simulink model "model_monocykl"  (R2014b)
settings: Solver=ode23  StartTime=0.0  StopTime=10.0  RelTol=1e-10
values from neighbouring files (symbols this model uses):
  k = 1    [astolfi.m]    (also in monocykl.m)
  p2 = -7    [astolfi.m]    (also in monocykl.m)
  p3 = 12    [astolfi.m]    (also in monocykl.m)
  teta0 = 0    [dynamika.m]    (also in kinematyka.m; monocykl.m = 3; wielomianowy.m)
  x0 = 0    [dynamika.m]    (also in kinematyka.m; monocykl.m = 4; wielomianowy.m = 1)
  y0 = 0    [dynamika.m]    (also in kinematyka.m; monocykl.m = 2; wielomianowy.m = 2)
settings Model: Creator=Dawid Perdek  LastModifiedBy=Dawid Perdek

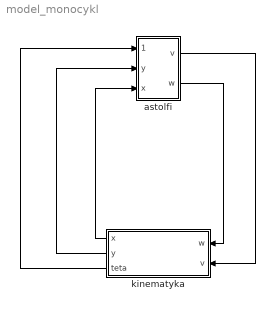
== system model_monocykl ==
  astolfi : Subsystem
  kinematyka : Subsystem
  wires:
  kinematyka/1(x) -> astolfi/3(x)
  kinematyka/2(y) -> astolfi/2(y)
  kinematyka/3(teta) -> astolfi/1(teta)
  astolfi/2(w) -> kinematyka/1(w)
  astolfi/1(v) -> kinematyka/2(v)

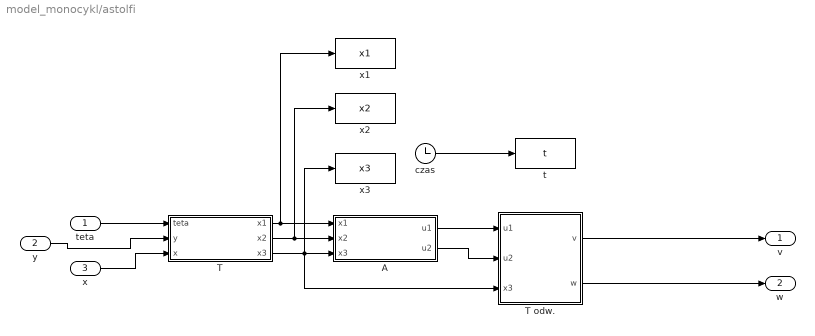
== system model_monocykl/astolfi ==
  teta : Inport
  y : Inport  Port=2
  x : Inport  Port=3
  A : Subsystem
  T : Subsystem
  T odw. : Subsystem
  czas : Clock
  t : ToWorkspace  VariableName=t  SampleTime=-1
  x1 : ToWorkspace  VariableName=x1  SampleTime=-1
  x2 : ToWorkspace  VariableName=x2  SampleTime=-1
  x3 : ToWorkspace  VariableName=x3  SampleTime=-1
  v : Outport
  w : Outport  Port=2
  wires:
  czas/1 -> t/1
  A/1(u1) -> T odw./1(u1)
  T/1(x1) -> x1/1, A/1(x1)
  T/3(x3) -> x3/1, T odw./3(x3), A/3(x3)
  A/2(u2) -> T odw./2(u2)
  T/2(x2) -> x2/1, A/2(x2)
  T odw./1(v) -> v/1
  T odw./2(w) -> w/1
  teta/1 -> T/1(teta)
  y/1 -> T/2(y)
  x/1 -> T/3(x)

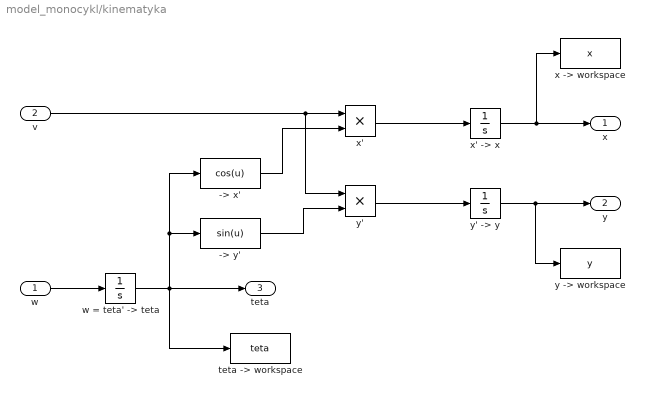
== system model_monocykl/kinematyka ==
  w : Inport
  v : Inport  Port=2
  -> x' : Fcn  Expr=cos(u)
  -> y' : Fcn  Expr=sin(u)
  "teta -> workspace" : ToWorkspace  VariableName=teta  SampleTime=-1
  "w = teta' -> teta" : Integrator  InitialCondition=teta0
  "x -> workspace" : ToWorkspace  VariableName=x  SampleTime=-1
  x' : Product
  "x' -> x" : Integrator  InitialCondition=x0
  "y -> workspace" : ToWorkspace  VariableName=y  SampleTime=-1
  y' : Product
  "y' -> y" : Integrator  InitialCondition=y0
  x : Outport
  y : Outport  Port=2
  teta : Outport  Port=3
  wires:
  w/1 -> "w = teta' -> teta"/1
  v/1 -> y'/1, x'/1
  -> x'/1 -> x'/2
  -> y'/1 -> y'/2
  x'/1 -> "x' -> x"/1
  y'/1 -> "y' -> y"/1
  "x' -> x"/1 -> "x -> workspace"/1, x/1
  "y' -> y"/1 -> "y -> workspace"/1, y/1
  "w = teta' -> teta"/1 -> "teta -> workspace"/1, -> x'/1, -> y'/1, teta/1

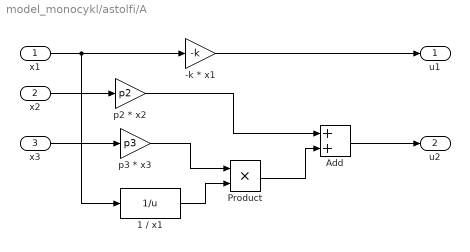
== system model_monocykl/astolfi/A ==
  x1 : Inport
  x2 : Inport  Port=2
  x3 : Inport  Port=3
  -k * x1 : Gain  Gain=-k
  1 / x1 : Fcn  Expr=1/u
  Add : Sum
  Product : Product
  p2 * x2 : Gain  Gain=p2
  p3 * x3 : Gain  Gain=p3
  u1 : Outport
  u2 : Outport  Port=2
  wires:
  p3 * x3/1 -> Product/1
  1 / x1/1 -> Product/2
  x1/1 -> 1 / x1/1, -k * x1/1
  x2/1 -> p2 * x2/1
  -k * x1/1 -> u1/1
  p2 * x2/1 -> Add/1
  x3/1 -> p3 * x3/1
  Add/1 -> u2/1
  Product/1 -> Add/2

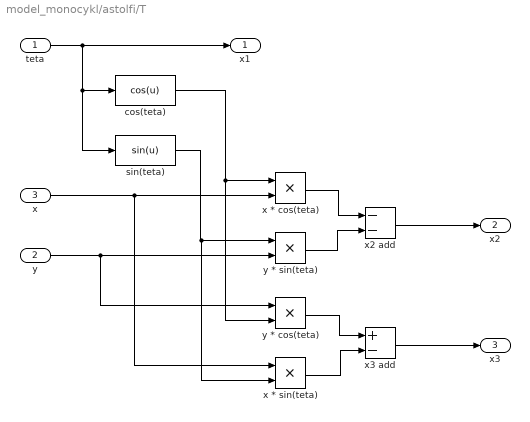
== system model_monocykl/astolfi/T ==
  teta : Inport
  y : Inport  Port=2
  x : Inport  Port=3
  cos(teta) : Fcn  Expr=cos(u)
  sin(teta) : Fcn  Expr=sin(u)
  x * cos(teta) : Product
  x * sin(teta) : Product
  x2 add : Sum  Inputs=--
  x3 add : Sum  Inputs=+-
  y * cos(teta) : Product
  y * sin(teta) : Product
  x1 : Outport
  x2 : Outport  Port=2
  x3 : Outport  Port=3
  wires:
  teta/1 -> sin(teta)/1, cos(teta)/1, x1/1
  cos(teta)/1 -> y * cos(teta)/2, x * cos(teta)/1
  x/1 -> x * sin(teta)/1, x * cos(teta)/2
  y/1 -> y * cos(teta)/1, y * sin(teta)/2
  sin(teta)/1 -> x * sin(teta)/2, y * sin(teta)/1
  x * cos(teta)/1 -> x2 add/1
  y * sin(teta)/1 -> x2 add/2
  y * cos(teta)/1 -> x3 add/1
  x * sin(teta)/1 -> x3 add/2
  x2 add/1 -> x2/1
  x3 add/1 -> x3/1

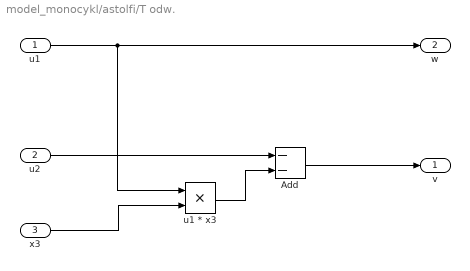
== system model_monocykl/astolfi/T odw. ==
  u1 : Inport
  u2 : Inport  Port=2
  x3 : Inport  Port=3
  Add : Sum  Inputs=--
  u1 * x3 : Product
  v : Outport
  w : Outport  Port=2
  wires:
  u1/1 -> w/1, u1 * x3/1
  x3/1 -> u1 * x3/2
  u1 * x3/1 -> Add/2
  u2/1 -> Add/1
  Add/1 -> v/1
